simulink model "LEO_MPC_SpeedCtrl"  (Simulink 9.3)
settings: Solver=ode45  StartTime=0.0  StopTime=100  RelTol=1e-3  EnableMultiTasking=on
libraries: Solver_SF x1
settings Model: Creator=admin  LastModifiedBy=梁秀华
settings DataIOCC: LimitDataPoints=on  SignalLoggingSaveFormat=Dataset
settings DebuggingCC: SolverPrmCheckMsg=warning  FcnCallInpInsideContextMsg=error
settings GRTTargetCC: GeneratePreprocessorConditionals=Disable all  CombineOutputUpdateFcns=on  GRTInterface=off

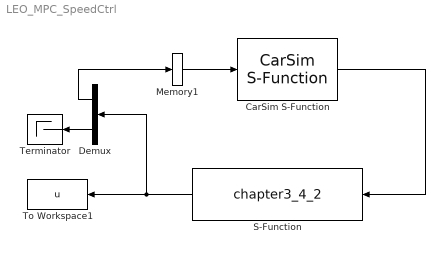
== system LEO_MPC_SpeedCtrl ==
  CarSim S-Function : Solver_SF/CarSim S-Function  Priority=1  SIMFILE=LEO_MPC_SpeedCtrl_du.sim
  Demux : Demux  Outputs=[2 4]
  Memory1 : Memory
  S-Function : S-Function  FunctionName=chapter3_4_2  SFunctionDeploymentMode=off  EnableBusSupport=off
  Terminator : Terminator
  To Workspace1 : ToWorkspace  VariableName=u  SaveFormat=Structure  SampleTime=-1
  wires:
  S-Function/1 -> Demux/1, To Workspace1/1
  Demux/1 -> Memory1/1
  Demux/2 -> Terminator/1
  CarSim S-Function/1 -> S-Function/1
  Memory1/1 -> CarSim S-Function/1
